simulink model "NetraAI_DigitalTwin_V2"  (Simulink 8.3)
settings: Solver=VariableStepDiscrete  StartTime=0.0  StopTime=1200  MaxStep=1  RelTol=1e-3
settings Model: Creator=kaustav  LastModifiedBy=kaustav
settings DataIOCC: SignalLoggingSaveFormat=Dataset
settings DebuggingCC: UnderspecifiedInitializationDetection=Simplified  StateNameClashWarn=none
settings GRTTargetCC: CombineOutputUpdateFcns=on  GRTInterface=off

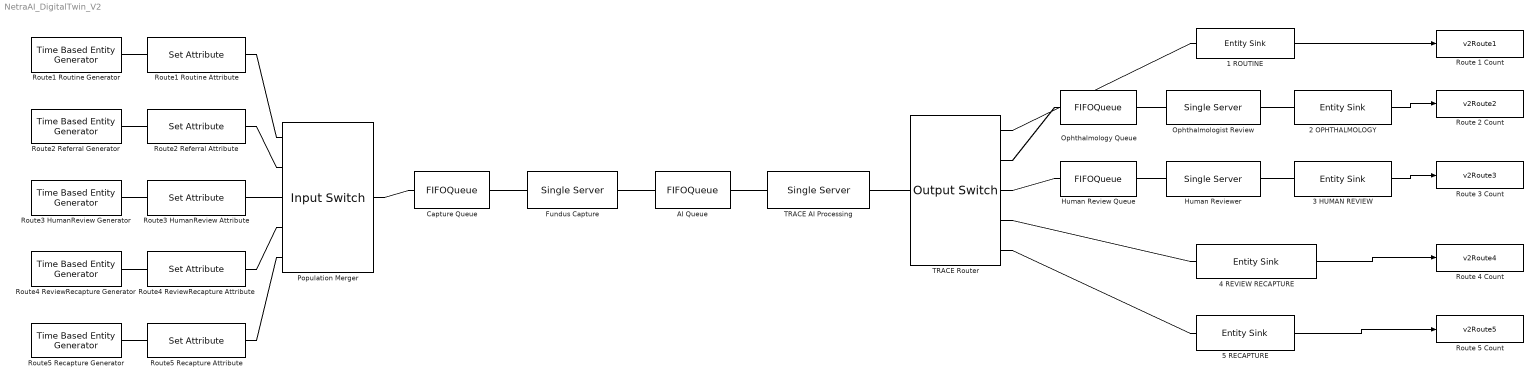
== system NetraAI_DigitalTwin_V2 ==
  1 ROUTINE : EntitySink  StatNumberArrived=on
  2 OPHTHALMOLOGY : EntitySink  StatNumberArrived=on
  3 HUMAN REVIEW : EntitySink  StatNumberArrived=on
  4 REVIEW RECAPTURE : EntitySink  StatNumberArrived=on
  5 RECAPTURE : EntitySink  StatNumberArrived=on
  AI Queue : FIFOQueue  Capacity=100
  Capture Queue : FIFOQueue  Capacity=100
  Fundus Capture : SingleServer  ServiceTime=12
  Human Review Queue : FIFOQueue  Capacity=100
  Human Reviewer : SingleServer  ServiceTime=45
  Ophthalmologist Review : SingleServer  ServiceTime=30
  Ophthalmology Queue : FIFOQueue  Capacity=100
  Population Merger : InputSwitch  NumberInputPorts=5
  Route 1 Count : ToWorkspace  VariableName=v2Route1  SampleTime=-1
  Route 2 Count : ToWorkspace  VariableName=v2Route2  SampleTime=-1
  Route 3 Count : ToWorkspace  VariableName=v2Route3  SampleTime=-1
  Route 4 Count : ToWorkspace  VariableName=v2Route4  SampleTime=-1
  Route 5 Count : ToWorkspace  VariableName=v2Route5  SampleTime=-1
  Route1 Routine Attribute : SetAttribute  AttributeName=routeCode  EvaluatedAttributeValue={ 1}
  Route1 Routine Generator : TimeBasedEntityGenerator  Period=75
  Route2 Referral Attribute : SetAttribute  AttributeName=routeCode  AttributeValue=2  EvaluatedAttributeValue={ 2}
  Route2 Referral Generator : TimeBasedEntityGenerator  Period=75
  Route3 HumanReview Attribute : SetAttribute  AttributeName=routeCode  AttributeValue=3  EvaluatedAttributeValue={ 3}
  Route3 HumanReview Generator : TimeBasedEntityGenerator  Period=75
  Route4 ReviewRecapture Attribute : SetAttribute  AttributeName=routeCode  AttributeValue=4  EvaluatedAttributeValue={ 4}
  Route4 ReviewRecapture Generator : TimeBasedEntityGenerator  Period=75
  Route5 Recapture Attribute : SetAttribute  AttributeName=routeCode  AttributeValue=5  EvaluatedAttributeValue={ 5}
  Route5 Recapture Generator : TimeBasedEntityGenerator  Period=75
  TRACE AI Processing : SingleServer  ServiceTime=8.67151
  TRACE Router : OutputSwitch  NumberOutputPorts=5  SwitchingCriterion=From attribute  AttributeName=routeCode
  wires:
  1 ROUTINE/1 -> Route 1 Count/1
  2 OPHTHALMOLOGY/1 -> Route 2 Count/1
  3 HUMAN REVIEW/1 -> Route 3 Count/1
  4 REVIEW RECAPTURE/1 -> Route 4 Count/1
  5 RECAPTURE/1 -> Route 5 Count/1
  connections:
  Route1 Routine Generator/RConn1 -- Route1 Routine Attribute/LConn1
  Route2 Referral Generator/RConn1 -- Route2 Referral Attribute/LConn1
  Route3 HumanReview Generator/RConn1 -- Route3 HumanReview Attribute/LConn1
  Route4 ReviewRecapture Generator/RConn1 -- Route4 ReviewRecapture Attribute/LConn1
  Route5 Recapture Generator/RConn1 -- Route5 Recapture Attribute/LConn1
  Route1 Routine Attribute/RConn1 -- Population Merger/LConn1
  Route2 Referral Attribute/RConn1 -- Population Merger/LConn2
  Route3 HumanReview Attribute/RConn1 -- Population Merger/LConn3
  Route4 ReviewRecapture Attribute/RConn1 -- Population Merger/LConn4
  Route5 Recapture Attribute/RConn1 -- Population Merger/LConn5
  Population Merger/RConn1 -- Capture Queue/LConn1
  Capture Queue/RConn1 -- Fundus Capture/LConn1
  Fundus Capture/RConn1 -- AI Queue/LConn1
  AI Queue/RConn1 -- TRACE AI Processing/LConn1
  TRACE AI Processing/RConn1 -- TRACE Router/LConn1
  TRACE Router/RConn1 -- 1 ROUTINE/LConn1
  TRACE Router/RConn2 -- Ophthalmology Queue/LConn1
  Ophthalmology Queue/RConn1 -- Ophthalmologist Review/LConn1
  Ophthalmologist Review/RConn1 -- 2 OPHTHALMOLOGY/LConn1
  TRACE Router/RConn3 -- Human Review Queue/LConn1
  Human Review Queue/RConn1 -- Human Reviewer/LConn1
  Human Reviewer/RConn1 -- 3 HUMAN REVIEW/LConn1
  TRACE Router/RConn4 -- 4 REVIEW RECAPTURE/LConn1
  TRACE Router/RConn5 -- 5 RECAPTURE/LConn1
